simulink model "rlKinovaBallBalance"  (R2024a)
settings: Solver=ode15s  StartTime=0.0  StopTime=200  RelTol=1e-3  AbsTol=1e-3
values from neighbouring files (symbols this model uses):
  max_torque = 0.75    [kinova_params.m]
  R1_q0 = 0    [kinova_params.m]
  R4_q0 = deg2rad(135)    [kinova_params.m]
  R5_q0 = 0    [kinova_params.m]
  rover_path = rover_path1    [mars_rover_params_all.m]
  U0 = [shoulder_torque_0 elbow_torque_0 wrist_torque_0 hand_torque_0]    [kinova_params.m]
undefined symbols (not defined in the file or in its folder): ball, Control, L1, L2, L3, LS1, LS3, plate, R1, R2, R3, Rover, RS1, RS3, X, Y, Z
libraries: sm_lib x256, nesl_utility x104, fl_lib x85, nesl_utility_internal x21, sdl_lib x20, ee_lib x10, mars_rover_lib x6, simulink x3, slpidlib x2, batteryecm_lib x2, robotalgslib x1, rllib x1
(part 6 of 11)

== system rlKinovaBallBalance/Kinova Ball Balance/Rover/Terrain/Contact ==
  Contact L1 : sm_lib/Forces and Torques/Spatial Contact Force  NormalForceType=SmoothSpringDamper  NormalStiffness=contact_k  NormalStiffnessUnits=N/m  NormalDamping=contact_d  NormalDampingUnits=N/(m/s)  NormalTransitionRegionWidth=contact_tw  NormalTransitionRegionWidthUnits=m  FrictionType=SmoothStickSlip  CoefficientOfStaticFriction=friction_mus  CoefficientOfDynamicFriction=friction_mud  FrictionalCriticalVelocity=friction_vcrit  FrictionalCriticalVelocityUnits=m/s  SenseContactSignal=off  SensePenetrationDepth=off  SenseSeparationDistance=off  SenseNormalForceMagnitude=off  SenseFrictionalForceMagnitude=off  SenseNormalVelocity=off  SenseTangentialVelocity=off  SenseContactBaseRotation=off  SenseContactBaseTranslation=off  SenseContactFollowerRotation=off  SenseContactFollowerTranslation=off  ZeroCrossDetectContactStartAndEnd=off
  Contact L2 : sm_lib/Forces and Torques/Spatial Contact Force  NormalForceType=SmoothSpringDamper  NormalStiffness=contact_k  NormalStiffnessUnits=N/m  NormalDamping=contact_d  NormalDampingUnits=N/(m/s)  NormalTransitionRegionWidth=contact_tw  NormalTransitionRegionWidthUnits=m  FrictionType=SmoothStickSlip  CoefficientOfStaticFriction=friction_mus  CoefficientOfDynamicFriction=friction_mud  FrictionalCriticalVelocity=friction_vcrit  FrictionalCriticalVelocityUnits=m/s  SenseContactSignal=off  SensePenetrationDepth=off  SenseSeparationDistance=off  SenseNormalForceMagnitude=off  SenseFrictionalForceMagnitude=off  SenseNormalVelocity=off  SenseTangentialVelocity=off  SenseContactBaseRotation=off  SenseContactBaseTranslation=off  SenseContactFollowerRotation=off  SenseContactFollowerTranslation=off  ZeroCrossDetectContactStartAndEnd=off
  Contact L3 : sm_lib/Forces and Torques/Spatial Contact Force  NormalForceType=SmoothSpringDamper  NormalStiffness=contact_k  NormalStiffnessUnits=N/m  NormalDamping=contact_d  NormalDampingUnits=N/(m/s)  NormalTransitionRegionWidth=contact_tw  NormalTransitionRegionWidthUnits=m  FrictionType=SmoothStickSlip  CoefficientOfStaticFriction=friction_mus  CoefficientOfDynamicFriction=friction_mud  FrictionalCriticalVelocity=friction_vcrit  FrictionalCriticalVelocityUnits=m/s  SenseContactSignal=off  SensePenetrationDepth=off  SenseSeparationDistance=off  SenseNormalForceMagnitude=off  SenseFrictionalForceMagnitude=off  SenseNormalVelocity=off  SenseTangentialVelocity=off  SenseContactBaseRotation=off  SenseContactBaseTranslation=off  SenseContactFollowerRotation=off  SenseContactFollowerTranslation=off  ZeroCrossDetectContactStartAndEnd=off
  Contact R1 : sm_lib/Forces and Torques/Spatial Contact Force  NormalForceType=SmoothSpringDamper  NormalStiffness=contact_k  NormalStiffnessUnits=N/m  NormalDamping=contact_d  NormalDampingUnits=N/(m/s)  NormalTransitionRegionWidth=contact_tw  NormalTransitionRegionWidthUnits=m  FrictionType=SmoothStickSlip  CoefficientOfStaticFriction=friction_mus  CoefficientOfDynamicFriction=friction_mud  FrictionalCriticalVelocity=friction_vcrit  FrictionalCriticalVelocityUnits=m/s  SenseContactSignal=off  SensePenetrationDepth=off  SenseSeparationDistance=off  SenseNormalForceMagnitude=off  SenseFrictionalForceMagnitude=off  SenseNormalVelocity=off  SenseTangentialVelocity=off  SenseContactBaseRotation=off  SenseContactBaseTranslation=off  SenseContactFollowerRotation=off  SenseContactFollowerTranslation=off  ZeroCrossDetectContactStartAndEnd=off
  Contact R2 : sm_lib/Forces and Torques/Spatial Contact Force  NormalForceType=SmoothSpringDamper  NormalStiffness=contact_k  NormalStiffnessUnits=N/m  NormalDamping=contact_d  NormalDampingUnits=N/(m/s)  NormalTransitionRegionWidth=contact_tw  NormalTransitionRegionWidthUnits=m  FrictionType=SmoothStickSlip  CoefficientOfStaticFriction=friction_mus  CoefficientOfDynamicFriction=friction_mud  FrictionalCriticalVelocity=friction_vcrit  FrictionalCriticalVelocityUnits=m/s  SenseContactSignal=off  SensePenetrationDepth=off  SenseSeparationDistance=off  SenseNormalForceMagnitude=off  SenseFrictionalForceMagnitude=off  SenseNormalVelocity=off  SenseTangentialVelocity=off  SenseContactBaseRotation=off  SenseContactBaseTranslation=off  SenseContactFollowerRotation=off  SenseContactFollowerTranslation=off  ZeroCrossDetectContactStartAndEnd=off
  Contact R3 : sm_lib/Forces and Torques/Spatial Contact Force  NormalForceType=SmoothSpringDamper  NormalStiffness=contact_k  NormalStiffnessUnits=N/m  NormalDamping=contact_d  NormalDampingUnits=N/(m/s)  NormalTransitionRegionWidth=contact_tw  NormalTransitionRegionWidthUnits=m  FrictionType=SmoothStickSlip  CoefficientOfStaticFriction=friction_mus  CoefficientOfDynamicFriction=friction_mud  FrictionalCriticalVelocity=friction_vcrit  FrictionalCriticalVelocityUnits=m/s  SenseContactSignal=off  SensePenetrationDepth=off  SenseSeparationDistance=off  SenseNormalForceMagnitude=off  SenseFrictionalForceMagnitude=off  SenseNormalVelocity=off  SenseTangentialVelocity=off  SenseContactBaseRotation=off  SenseContactBaseTranslation=off  SenseContactFollowerRotation=off  SenseContactFollowerTranslation=off  ZeroCrossDetectContactStartAndEnd=off
  Simscape Bus : SimscapeBus  HierarchyStrings=L1;L2;L3;R1;R2;R3
  Wheels : PMIOPort  Side=Right
  Surface : PMIOPort  Port=2  Side=Right
  connections:
  Contact R2/RConn1 -- Simscape Bus/LConn5
  Contact L2/RConn1 -- Simscape Bus/LConn2
  Contact L1/LConn1 -- Contact L2/LConn1 -- Contact L3/LConn1 -- Surface/RConn1 -- Contact R1/LConn1 -- Contact R3/LConn1 -- Contact R2/LConn1
  Contact L1/RConn1 -- Simscape Bus/LConn1
  Contact R3/RConn1 -- Simscape Bus/LConn6
  Simscape Bus/RConn1 -- Wheels/RConn1
  Contact R1/RConn1 -- Simscape Bus/LConn4
  Contact L3/RConn1 -- Simscape Bus/LConn3

== system rlKinovaBallBalance/Kinova Ball Balance/7 DOF Manipulator/Bracelet_Link/Bracelet Link/FileSolid ==
  Bracelet Link : sm_lib/Body Elements/File Solid  ExtGeomFileName=bracelet_with_vision_link.STL  UnitType=Custom  ExtGeomFileUnits=m  StepReaderType=HEX  ExportConvexHullGeometry=off  InertiaType=Custom  BasedOnType=DensityFromFile  Density=1000  DensityUnits=kg/m^3  Mass=0.0639903  MassUnits=kg  CenterOfMass=[-0.000374733, 0.0200972, 0.0397002]  CenterOfMassUnits=m  MomentsOfInertia=[8.77763e-05, 5.386e-05, 0.000111032]  MomentsOfInertiaUnits=kg*m^2  ProductsOfInertia=[-7.81917e-06, 1.77829e-07, -4.01652e-07]  ProductsOfInertiaUnits=kg*m^2  GraphicType=FromGeometry  MarkerShape=Sphere  MarkerSize=10  GraphicVisPropType=SimpleVisualProperties  GraphicDiffuseColor=[0.6666667 0.77254903 0.92941177]  GraphicOpacity=1  GraphicSpecularColor=[0.5 0.5 0.5 1.0]  GraphicAmbientColor=[0.15 0.15 0.15 1.0]  GraphicEmissiveColor=[0.0 0.0 0.0 1.0]  GraphicShininess=75  DoExposeReferenceFrame=on  SerializedFrames=<Frames/>
  R : PMIOPort  Side=Right
  connections:
  Bracelet Link/RConn1 -- R/RConn1

== system rlKinovaBallBalance/Kinova Ball Balance/7 DOF Manipulator/Bracelet_Link/Bracelet Link/Inertia ==
  Inertia1 : sm_lib/Body Elements/Inertia  InertiaType=Custom  Mass=0.0639903  MassUnits=kg  CenterOfMass=[-0.000374733, 0.0200972, 0.0397002]  CenterOfMassUnits=m  MomentsOfInertia=[8.77763e-05, 5.386e-05, 0.000111032]  MomentsOfInertiaUnits=kg*m^2  ProductsOfInertia=[-7.81917e-06, 1.77829e-07, -4.01652e-07]  ProductsOfInertiaUnits=kg*m^2  GraphicType=Marker  MarkerShape=Inertia  MarkerSize=20  GraphicVisPropType=SimpleVisualProperties  GraphicDiffuseColor=[0.5 0.5 0.5]  GraphicOpacity=1.0  GraphicSpecularColor=[0.5 0.5 0.5 1.0]  GraphicAmbientColor=[0.15 0.15 0.15 1.0]  GraphicEmissiveColor=[0.0 0.0 0.0 1.0]  GraphicShininess=75
  R : PMIOPort  Side=Right
  connections:
  Inertia1/RConn1 -- R/RConn1

== system rlKinovaBallBalance/Kinova Ball Balance/7 DOF Manipulator/ForeArm_Link/ForeArm Link/FileSolid ==
  Forearm Link : sm_lib/Body Elements/File Solid  ExtGeomFileName=forearm_link.STL  UnitType=Custom  ExtGeomFileUnits=m  StepReaderType=HEX  ExportConvexHullGeometry=off  InertiaType=Custom  BasedOnType=DensityFromFile  Density=1000  DensityUnits=kg/m^3  Mass=0.108759  MassUnits=kg  CenterOfMass=[0.0794976, 0.0148416, -8.39544e-07]  CenterOfMassUnits=m  MomentsOfInertia=[0.000118324, 0.000832188, 0.000809477]  MomentsOfInertiaUnits=kg*m^2  ProductsOfInertia=[3.60538e-09, -2.24072e-09, 7.50733e-05]  ProductsOfInertiaUnits=kg*m^2  GraphicType=FromGeometry  MarkerShape=Sphere  MarkerSize=10  GraphicVisPropType=SimpleVisualProperties  GraphicDiffuseColor=[0.54509807 0.654902 0.77254903]  GraphicOpacity=1  GraphicSpecularColor=[0.5 0.5 0.5 1.0]  GraphicAmbientColor=[0.15 0.15 0.15 1.0]  GraphicEmissiveColor=[0.0 0.0 0.0 1.0]  GraphicShininess=75  DoExposeReferenceFrame=on  SerializedFrames=<Frames/>
  R : PMIOPort  Side=Right
  connections:
  Forearm Link/RConn1 -- R/RConn1

== system rlKinovaBallBalance/Kinova Ball Balance/7 DOF Manipulator/ForeArm_Link/ForeArm Link/Inertia ==
  Inertia1 : sm_lib/Body Elements/Inertia  InertiaType=Custom  Mass=0.108759  MassUnits=kg  CenterOfMass=[0.0794976, 0.0148416, -8.39544e-07]  CenterOfMassUnits=m  MomentsOfInertia=[0.000118324, 0.000832188, 0.000809477]  MomentsOfInertiaUnits=kg*m^2  ProductsOfInertia=[3.60538e-09, -2.24072e-09, 7.50733e-05]  ProductsOfInertiaUnits=kg*m^2  GraphicType=Marker  MarkerShape=Inertia  MarkerSize=20  GraphicVisPropType=SimpleVisualProperties  GraphicDiffuseColor=[0.5 0.5 0.5]  GraphicOpacity=1.0  GraphicSpecularColor=[0.5 0.5 0.5 1.0]  GraphicAmbientColor=[0.15 0.15 0.15 1.0]  GraphicEmissiveColor=[0.0 0.0 0.0 1.0]  GraphicShininess=75
  R : PMIOPort  Side=Right
  connections:
  Inertia1/RConn1 -- R/RConn1

== system rlKinovaBallBalance/Kinova Ball Balance/7 DOF Manipulator/HalfArm1_Link/HalfArm1 Link/FileSolid ==
  Half Arm1 Link : sm_lib/Body Elements/File Solid  ExtGeomFileName=half_arm_1_link.STL  UnitType=Custom  ExtGeomFileUnits=m  StepReaderType=HEX  ExportConvexHullGeometry=off  InertiaType=Custom  BasedOnType=DensityFromFile  Density=1000  DensityUnits=kg/m^3  Mass=0.137977  MassUnits=kg  CenterOfMass=[0.100808, 0.0121234, 4.10274e-06]  CenterOfMassUnits=m  MomentsOfInertia=[0.000202425, 0.00113112, 0.00110619]  MomentsOfInertiaUnits=kg*m^2  ProductsOfInertia=[1.72409e-08, -8.98835e-09, 0.000105223]  ProductsOfInertiaUnits=kg*m^2  GraphicType=FromGeometry  MarkerShape=Sphere  MarkerSize=10  GraphicVisPropType=SimpleVisualProperties  GraphicDiffuseColor=[0.54509807 0.654902 0.77254903]  GraphicOpacity=1  GraphicSpecularColor=[0.5 0.5 0.5 1.0]  GraphicAmbientColor=[0.15 0.15 0.15 1.0]  GraphicEmissiveColor=[0.0 0.0 0.0 1.0]  GraphicShininess=75  DoExposeReferenceFrame=on  SerializedFrames=<Frames/>
  R : PMIOPort  Side=Right
  connections:
  Half Arm1 Link/RConn1 -- R/RConn1

== system rlKinovaBallBalance/Kinova Ball Balance/7 DOF Manipulator/HalfArm1_Link/HalfArm1 Link/Inertia ==
  Inertia1 : sm_lib/Body Elements/Inertia  InertiaType=Custom  Mass=0.137977  MassUnits=kg  CenterOfMass=[0.100808, 0.0121234, 4.10274e-06]  CenterOfMassUnits=m  MomentsOfInertia=[0.000202425, 0.00113112, 0.00110619]  MomentsOfInertiaUnits=kg*m^2  ProductsOfInertia=[1.72409e-08, -8.98835e-09, 0.000105223]  ProductsOfInertiaUnits=kg*m^2  GraphicType=Marker  MarkerShape=Inertia  MarkerSize=20  GraphicVisPropType=SimpleVisualProperties  GraphicDiffuseColor=[0.5 0.5 0.5]  GraphicOpacity=1.0  GraphicSpecularColor=[0.5 0.5 0.5 1.0]  GraphicAmbientColor=[0.15 0.15 0.15 1.0]  GraphicEmissiveColor=[0.0 0.0 0.0 1.0]  GraphicShininess=75
  R : PMIOPort  Side=Right
  connections:
  Inertia1/RConn1 -- R/RConn1

== system rlKinovaBallBalance/Kinova Ball Balance/7 DOF Manipulator/HalfArm2_Link/HalfArm2 Link/FileSolid ==
  Half Arm2 Link : sm_lib/Body Elements/File Solid  ExtGeomFileName=half_arm_2_link.STL  UnitType=Custom  ExtGeomFileUnits=m  StepReaderType=HEX  ExportConvexHullGeometry=off  InertiaType=Custom  BasedOnType=DensityFromFile  Density=1000  DensityUnits=kg/m^3  Mass=0.137978  MassUnits=kg  CenterOfMass=[0.0871838, 0.0118108, 4.16659e-06]  CenterOfMassUnits=m  MomentsOfInertia=[0.000195075, 0.0011006, 0.00106833]  MomentsOfInertiaUnits=kg*m^2  ProductsOfInertia=[1.66656e-08, -1.69023e-08, 7.86653e-05]  ProductsOfInertiaUnits=kg*m^2  GraphicType=FromGeometry  MarkerShape=Sphere  MarkerSize=10  GraphicVisPropType=SimpleVisualProperties  GraphicDiffuseColor=[0.6666667 0.77254903 0.92941177]  GraphicOpacity=1  GraphicSpecularColor=[0.5 0.5 0.5 1.0]  GraphicAmbientColor=[0.15 0.15 0.15 1.0]  GraphicEmissiveColor=[0.0 0.0 0.0 1.0]  GraphicShininess=75  DoExposeReferenceFrame=on  SerializedFrames=<Frames/>
  R : PMIOPort  Side=Right
  connections:
  Half Arm2 Link/RConn1 -- R/RConn1

== system rlKinovaBallBalance/Kinova Ball Balance/7 DOF Manipulator/HalfArm2_Link/HalfArm2 Link/Inertia ==
  Inertia1 : sm_lib/Body Elements/Inertia  InertiaType=Custom  Mass=0.137978  MassUnits=kg  CenterOfMass=[0.0871838, 0.0118108, 4.16659e-06]  CenterOfMassUnits=m  MomentsOfInertia=[0.000195075, 0.0011006, 0.00106833]  MomentsOfInertiaUnits=kg*m^2  ProductsOfInertia=[1.66656e-08, -1.69023e-08, 7.86653e-05]  ProductsOfInertiaUnits=kg*m^2  GraphicType=Marker  MarkerShape=Inertia  MarkerSize=20  GraphicVisPropType=SimpleVisualProperties  GraphicDiffuseColor=[0.5 0.5 0.5]  GraphicOpacity=1.0  GraphicSpecularColor=[0.5 0.5 0.5 1.0]  GraphicAmbientColor=[0.15 0.15 0.15 1.0]  GraphicEmissiveColor=[0.0 0.0 0.0 1.0]  GraphicShininess=75
  R : PMIOPort  Side=Right
  connections:
  Inertia1/RConn1 -- R/RConn1

== system rlKinovaBallBalance/Kinova Ball Balance/7 DOF Manipulator/Shoulder_Link/Shoulder Link/FileSolid ==
  Shoulder Link : sm_lib/Body Elements/File Solid  ExtGeomFileName=shoulder_link.STL  UnitType=Custom  ExtGeomFileUnits=m  StepReaderType=HEX  ExportConvexHullGeometry=off  InertiaType=Custom  BasedOnType=DensityFromFile  Density=1000  DensityUnits=kg/m^3  Mass=0.206679  MassUnits=kg  CenterOfMass=[0.0758362, 0.0170163, 7.48345e-07]  CenterOfMassUnits=m  MomentsOfInertia=[0.000301623, 0.000658228, 0.000584422]  MomentsOfInertiaUnits=kg*m^2  ProductsOfInertia=[6.12368e-09, 4.93274e-09, -6.36892e-05]  ProductsOfInertiaUnits=kg*m^2  GraphicType=FromGeometry  MarkerShape=Sphere  MarkerSize=10  GraphicVisPropType=SimpleVisualProperties  GraphicDiffuseColor=[0.6666667 0.77254903 0.92941177]  GraphicOpacity=1  GraphicSpecularColor=[0.5 0.5 0.5 1.0]  GraphicAmbientColor=[0.15 0.15 0.15 1.0]  GraphicEmissiveColor=[0.0 0.0 0.0 1.0]  GraphicShininess=75  DoExposeReferenceFrame=on  SerializedFrames=<Frames/>
  R : PMIOPort  Side=Right
  connections:
  R/RConn1 -- Shoulder Link/RConn1

== system rlKinovaBallBalance/Kinova Ball Balance/7 DOF Manipulator/Shoulder_Link/Shoulder Link/Inertia ==
  Inertia1 : sm_lib/Body Elements/Inertia  InertiaType=Custom  Mass=0.206679  MassUnits=kg  CenterOfMass=[0.0758362, 0.0170163, 7.48345e-07]  CenterOfMassUnits=m  MomentsOfInertia=[0.000301623, 0.000658228, 0.000584422]  MomentsOfInertiaUnits=kg*m^2  ProductsOfInertia=[6.12368e-09, 4.93274e-09, -6.36892e-05]  ProductsOfInertiaUnits=kg*m^2  GraphicType=Marker  MarkerShape=Inertia  MarkerSize=20  GraphicVisPropType=SimpleVisualProperties  GraphicDiffuseColor=[0.5 0.5 0.5]  GraphicOpacity=1.0  GraphicSpecularColor=[0.5 0.5 0.5 1.0]  GraphicAmbientColor=[0.15 0.15 0.15 1.0]  GraphicEmissiveColor=[0.0 0.0 0.0 1.0]  GraphicShininess=75
  R : PMIOPort  Side=Right
  connections:
  Inertia1/RConn1 -- R/RConn1

== system rlKinovaBallBalance/Kinova Ball Balance/7 DOF Manipulator/Wrist1_Link/Wrist1 Link/FileSolid ==
  Wrist1 Link : sm_lib/Body Elements/File Solid  ExtGeomFileName=spherical_wrist_1_link.STL  UnitType=Custom  ExtGeomFileUnits=m  StepReaderType=HEX  ExportConvexHullGeometry=off  InertiaType=Custom  BasedOnType=DensityFromFile  Density=1000  DensityUnits=kg/m^3  Mass=0.0607261  MassUnits=kg  CenterOfMass=[0.0669267, 0.0134734, -3.64177e-07]  CenterOfMassUnits=m  MomentsOfInertia=[5.88928e-05, 0.000140521, 0.000138155]  MomentsOfInertiaUnits=kg*m^2  ProductsOfInertia=[2.83121e-09, 1.56006e-09, -2.20674e-05]  ProductsOfInertiaUnits=kg*m^2  GraphicType=FromGeometry  MarkerShape=Sphere  MarkerSize=10  GraphicVisPropType=SimpleVisualProperties  GraphicDiffuseColor=[0.6666667 0.77254903 0.92941177]  GraphicOpacity=1  GraphicSpecularColor=[0.5 0.5 0.5 1.0]  GraphicAmbientColor=[0.15 0.15 0.15 1.0]  GraphicEmissiveColor=[0.0 0.0 0.0 1.0]  GraphicShininess=75  DoExposeReferenceFrame=on  SerializedFrames=<Frames/>
  R : PMIOPort  Side=Right
  connections:
  Wrist1 Link/RConn1 -- R/RConn1

== system rlKinovaBallBalance/Kinova Ball Balance/7 DOF Manipulator/Wrist1_Link/Wrist1 Link/Inertia ==
  Inertia1 : sm_lib/Body Elements/Inertia  InertiaType=Custom  Mass=0.0607261  MassUnits=kg  CenterOfMass=[0.0669267, 0.0134734, -3.64177e-07]  CenterOfMassUnits=m  MomentsOfInertia=[5.88928e-05, 0.000140521, 0.000138155]  MomentsOfInertiaUnits=kg*m^2  ProductsOfInertia=[2.83121e-09, 1.56006e-09, -2.20674e-05]  ProductsOfInertiaUnits=kg*m^2  GraphicType=Marker  MarkerShape=Inertia  MarkerSize=20  GraphicVisPropType=SimpleVisualProperties  GraphicDiffuseColor=[0.5 0.5 0.5]  GraphicOpacity=1.0  GraphicSpecularColor=[0.5 0.5 0.5 1.0]  GraphicAmbientColor=[0.15 0.15 0.15 1.0]  GraphicEmissiveColor=[0.0 0.0 0.0 1.0]  GraphicShininess=75
  R : PMIOPort  Side=Right
  connections:
  Inertia1/RConn1 -- R/RConn1

== system rlKinovaBallBalance/Kinova Ball Balance/7 DOF Manipulator/Wrist2_Link/Wrist2 Link/FileSolid ==
  Wrist2 Link : sm_lib/Body Elements/File Solid  ExtGeomFileName=spherical_wrist_2_link.STL  UnitType=Custom  ExtGeomFileUnits=m  StepReaderType=HEX  ExportConvexHullGeometry=off  InertiaType=Custom  BasedOnType=DensityFromFile  Density=1000  DensityUnits=kg/m^3  Mass=0.0607235  MassUnits=kg  CenterOfMass=[0.0566892, 0.0133552, 2.07599e-07]  CenterOfMassUnits=m  MomentsOfInertia=[6.22269e-05, 0.000150545, 0.000151516]  MomentsOfInertiaUnits=kg*m^2  ProductsOfInertia=[-8.5602e-09, -1.23542e-08, -3.01223e-05]  ProductsOfInertiaUnits=kg*m^2  GraphicType=FromGeometry  MarkerShape=Sphere  MarkerSize=10  GraphicVisPropType=SimpleVisualProperties  GraphicDiffuseColor=[0.54509807 0.654902 0.77254903]  GraphicOpacity=1  GraphicSpecularColor=[0.5 0.5 0.5 1.0]  GraphicAmbientColor=[0.15 0.15 0.15 1.0]  GraphicEmissiveColor=[0.0 0.0 0.0 1.0]  GraphicShininess=75  DoExposeReferenceFrame=on  SerializedFrames=<Frames/>
  R : PMIOPort  Side=Right
  connections:
  Wrist2 Link/RConn1 -- R/RConn1

== system rlKinovaBallBalance/Kinova Ball Balance/7 DOF Manipulator/Wrist2_Link/Wrist2 Link/Inertia ==
  Inertia1 : sm_lib/Body Elements/Inertia  InertiaType=Custom  Mass=0.0607235  MassUnits=kg  CenterOfMass=[0.0566892, 0.0133552, 2.07599e-07]  CenterOfMassUnits=m  MomentsOfInertia=[6.22269e-05, 0.000150545, 0.000151516]  MomentsOfInertiaUnits=kg*m^2  ProductsOfInertia=[-8.5602e-09, -1.23542e-08, -3.01223e-05]  ProductsOfInertiaUnits=kg*m^2  GraphicType=Marker  MarkerShape=Inertia  MarkerSize=20  GraphicVisPropType=SimpleVisualProperties  GraphicDiffuseColor=[0.5 0.5 0.5]  GraphicOpacity=1.0  GraphicSpecularColor=[0.5 0.5 0.5 1.0]  GraphicAmbientColor=[0.15 0.15 0.15 1.0]  GraphicEmissiveColor=[0.0 0.0 0.0 1.0]  GraphicShininess=75
  R : PMIOPort  Side=Right
  connections:
  Inertia1/RConn1 -- R/RConn1

== system rlKinovaBallBalance/Kinova Ball Balance/7 DOF Manipulator/base_link/Base Link/FileSolid ==
  Base Link : sm_lib/Body Elements/File Solid  ExtGeomFileName=base_link.STL  UnitType=Custom  ExtGeomFileUnits=m  StepReaderType=HEX  ExportConvexHullGeometry=off  InertiaType=Custom  BasedOnType=DensityFromFile  Density=1000  DensityUnits=kg/m^3  Mass=1.06185  MassUnits=kg  CenterOfMass=[0.000712614, 0.0763467, 0.000106583]  CenterOfMassUnits=m  MomentsOfInertia=[0.00275492, 0.0011525, 0.00277912]  MomentsOfInertiaUnits=kg*m^2  ProductsOfInertia=[-1.84082e-06, 1.0557e-07, 2.81404e-05]  ProductsOfInertiaUnits=kg*m^2  GraphicType=FromGeometry  MarkerShape=Sphere  MarkerSize=10  GraphicVisPropType=SimpleVisualProperties  GraphicDiffuseColor=[0.54509807 0.654902 0.77254903]  GraphicOpacity=1  GraphicSpecularColor=[0.5 0.5 0.5 1.0]  GraphicAmbientColor=[0.15 0.15 0.15 1.0]  GraphicEmissiveColor=[0.0 0.0 0.0 1.0]  GraphicShininess=75  DoExposeReferenceFrame=on  SerializedFrames=<Frames/>
  R : PMIOPort  Side=Right
  connections:
  Base Link/RConn1 -- R/RConn1

== system rlKinovaBallBalance/Kinova Ball Balance/7 DOF Manipulator/base_link/Base Link/Inertia ==
  Inertia : sm_lib/Body Elements/Inertia  InertiaType=Custom  Mass=1.06185  MassUnits=kg  CenterOfMass=[0.000712614, 0.0763467, 0.000106583]  CenterOfMassUnits=m  MomentsOfInertia=[0.00275492, 0.0011525, 0.00277912]  MomentsOfInertiaUnits=kg*m^2  ProductsOfInertia=[-1.84082e-06, 1.0557e-07, 2.81404e-05]  ProductsOfInertiaUnits=kg*m^2  GraphicType=Marker  MarkerShape=Inertia  MarkerSize=20  GraphicVisPropType=SimpleVisualProperties  GraphicDiffuseColor=[0.5 0.5 0.5]  GraphicOpacity=1.0  GraphicSpecularColor=[0.5 0.5 0.5 1.0]  GraphicAmbientColor=[0.15 0.15 0.15 1.0]  GraphicEmissiveColor=[0.0 0.0 0.0 1.0]  GraphicShininess=75
  R : PMIOPort  Side=Right
  connections:
  Inertia/RConn1 -- R/RConn1

== system rlKinovaBallBalance/Kinova Ball Balance/Control/Chassis Control/Ackerman Steer Angle/Hold Steer at Goal ==
  d : Inport
  Enable : EnablePort
  d_h : Outport
  wires:
  d/1 -> d_h/1

== system rlKinovaBallBalance/Kinova Ball Balance/Control/Chassis Control/Steering Controller/Bus to Vec ==
  B : Inport
  Bus Selector : BusSelector  OutputSignals=q.L3,q.L1,q.R3,q.R1
  Mux : Mux
  V : Outport
  wires:
  Bus Selector/1 -> Mux/1  "<L3>"
  Bus Selector/4 -> Mux/4  "<R1>"
  Mux/1 -> V/1
  Bus Selector/2 -> Mux/2  "<L1>"
  Bus Selector/3 -> Mux/3  "<R3>"
  B/1 -> Bus Selector/1

== system rlKinovaBallBalance/Kinova Ball Balance/Control/Chassis Control/Steering Controller/Check Difference ==
  tgt : Inport
  meas : Inport  Port=2
  Demux1 : Demux
  Demux2 : Demux
  Mux{,1..3} (4 alike) : Mux  Inputs=2
  L3 : Outport
  L1 : Outport  Port=2
  R3 : Outport  Port=3
  R1 : Outport  Port=4
  wires:
  Demux2/1 -> Mux/2
  Demux1/3 -> Mux2/1
  Demux1/2 -> Mux1/1
  Demux2/4 -> Mux3/2
  Demux2/2 -> Mux1/2
  Demux2/3 -> Mux2/2
  meas/1 -> Demux2/1
  Demux1/1 -> Mux/1
  Mux1/1 -> L1/1
  Demux1/4 -> Mux3/1
  Mux3/1 -> R1/1
  Mux2/1 -> R3/1
  Mux/1 -> L3/1
  tgt/1 -> Demux1/1

== system rlKinovaBallBalance/Kinova Ball Balance/Control/Chassis Control/Steering Controller/Filter qMeas ==
  In : Inport
  Gain : Gain  Gain=1./b
  Integrator : Integrator  InitialCondition=x_initial.*b
  Sum : Sum  Inputs=|+-  InputSameDT=on  SaturateOnIntegerOverflow=on  OutDataTypeStr=Inherit: Same as first input
  Out : Outport  VectorParamsAs1DForOutWhenUnconnected=off
  wires:
  Sum/1 -> Integrator/1
  In/1 -> Sum/1
  Integrator/1 -> Gain/1
  Gain/1 -> Sum/2, Out/1

== system rlKinovaBallBalance/Kinova Ball Balance/Control/Chassis Control/Steering Controller/Filter qTarget ==
  In : Inport
  Gain : Gain  Gain=1./b
  Integrator : Integrator  InitialCondition=x_initial.*b
  Sum : Sum  Inputs=|+-  InputSameDT=on  SaturateOnIntegerOverflow=on  OutDataTypeStr=Inherit: Same as first input
  Out : Outport  VectorParamsAs1DForOutWhenUnconnected=off
  wires:
  Gain/1 -> Out/1, Sum/2
  Integrator/1 -> Gain/1
  In/1 -> Sum/1
  Sum/1 -> Integrator/1

== system rlKinovaBallBalance/Kinova Ball Balance/Control/Chassis Control/Target Direction and Speed/Check Distance To Goal ==
  note: Distance from Goal to satisfy that the robot has reached the goal
  goal : Inport
  currentPose : Inport  Port=2
  linVel : Inport  Port=3
  Add : Sum
  Constant : Constant  Value=0.25
  Constant1 : Constant  Value=2*Control.Drive.TargetAccel
  Divide : Product  Inputs=*/
  Dot Product : DotProduct  OutDataTypeStr=Inherit: Inherit via internal rule
  Gain1 : Gain
  Less Than : RelationalOperator  Operator=>  OutDataTypeStr=boolean  RndMeth=Simplest  InputSameDT=off
  Less Than1 : RelationalOperator  Operator=>  OutDataTypeStr=boolean  RndMeth=Simplest  InputSameDT=off
  NOT : Logic  Operator=NOT  IconShape=distinctive  AllPortsSameDT=off  OutDataTypeStr=boolean
  Scope1 : Scope
  Selector : Selector  InputPortWidth=3  IndexOptions=Index vector (dialog)  Indices=[1 2]  OutputSizes=1
  Sqrt : Sqrt
  Subtract : Sum  Inputs=+-
  Unit Delay : UnitDelay  SampleTime=-1  HasFrameUpgradeWarning=on
  const : Math  Operator=square
  atGoal : Outport
  Slow : Outport  Port=2
  wires:
  goal/1 -> Subtract/2
  Dot Product/1 -> Sqrt/1
  Constant/1 -> Gain1/1, Less Than/2
  currentPose/1 -> Selector/1
  Sqrt/1 -> Scope1/1, Less Than/1, Less Than1/1
  Subtract/1 -> Dot Product/2, Dot Product/1
  Selector/1 -> Subtract/1
  linVel/1 -> const/1
  const/1 -> Divide/1
  Constant1/1 -> Divide/2
  Less Than1/1 -> Slow/1
  Add/1 -> Less Than1/2
  Divide/1 -> Add/1
  Gain1/1 -> Add/2
  Less Than/1 -> NOT/1
  NOT/1 -> Unit Delay/1
  Unit Delay/1 -> atGoal/1

== system rlKinovaBallBalance/Kinova Ball Balance/Control/Chassis Control/Target Direction and Speed/hold ==
  In1 : Inport
  Constant9 : Constant  Value=inf
  NOT1 : Logic  Operator=NOT  IconShape=distinctive  AllPortsSameDT=off  OutDataTypeStr=boolean
  RoverStopTime : Subsystem
  Switch3 : Switch  Criteria=u2 > Threshold  SaturateOnIntegerOverflow=off  InputSameDT=off
  Unit Delay1 : UnitDelay  SampleTime=-1  HasFrameUpgradeWarning=on
  Out1 : Outport
  wires:
  Unit Delay1/1 -> Switch3/2
  RoverStopTime/1(DeAccelTime) -> Switch3/1
  Switch3/1 -> Out1/1
  NOT1/1 -> RoverStopTime/1(Enable), Unit Delay1/1
  Constant9/1 -> Switch3/3
  In1/1 -> NOT1/1

== system rlKinovaBallBalance/Kinova Ball Balance/Control/Chassis Control/Wheel Speed Controller/Bus to Vec ==
  B : Inport
  Bus Selector : BusSelector  OutputSignals=w.L1,w.L2,w.L3,w.R1,w.R2,w.R3
  Mux : Mux  Inputs=6
  V : Outport
  wires:
  Bus Selector/1 -> Mux/1  "<L1>"
  Bus Selector/3 -> Mux/3  "<L3>"
  Bus Selector/4 -> Mux/4  "<R1>"
  Bus Selector/6 -> Mux/6  "<R3>"
  Bus Selector/5 -> Mux/5  "<R2>"
  Bus Selector/2 -> Mux/2  "<L2>"
  B/1 -> Bus Selector/1
  Mux/1 -> V/1

== system rlKinovaBallBalance/Kinova Ball Balance/Control/Chassis Control/Wheel Speed Controller/Filter wMeas ==
  In : Inport
  Gain : Gain  Gain=1./b
  Integrator : Integrator  InitialCondition=x_initial.*b
  Sum : Sum  Inputs=|+-  InputSameDT=on  SaturateOnIntegerOverflow=on  OutDataTypeStr=Inherit: Same as first input
  Out : Outport  VectorParamsAs1DForOutWhenUnconnected=off
  wires:
  Sum/1 -> Integrator/1
  In/1 -> Sum/1
  Integrator/1 -> Gain/1
  Gain/1 -> Sum/2, Out/1

== system rlKinovaBallBalance/Kinova Ball Balance/Control/Chassis Control/Wheel Speed Controller/Filter wTarget ==
  In : Inport
  Gain : Gain  Gain=1./b
  Integrator : Integrator  InitialCondition=x_initial.*b
  Sum : Sum  Inputs=|+-  InputSameDT=on  SaturateOnIntegerOverflow=on  OutDataTypeStr=Inherit: Same as first input
  Out : Outport  VectorParamsAs1DForOutWhenUnconnected=off
  wires:
  Gain/1 -> Out/1, Sum/2
  Integrator/1 -> Gain/1
  In/1 -> Sum/1
  Sum/1 -> Integrator/1

== system rlKinovaBallBalance/Kinova Ball Balance/Rover/Chassis/Camera/rsm_base_1_RIGID ==
  ReferenceFrame : sm_lib/Frames and Transforms/Reference Frame
  Solid : sm_lib/Body Elements/File Solid  ExtGeomFileName=rover_chassis_sensor_base.stl  UnitType=Custom  ExtGeomFileUnits=cm  StepReaderType=HEX  ExportConvexHullGeometry=off  InertiaType=CalculateFromGeometry  BasedOnType=Density  Density=2000  DensityUnits=kg/m^3  Mass=202690.508551217  MassUnits=kg  CenterOfMass=[-2.09994238818055e-07 21.8231915316941 -2.20167989735098e-07]  CenterOfMassUnits=m  MomentsOfInertia=[2411866.97125594 5940029.20050206 6701187.74240286]  MomentsOfInertiaUnits=kg*m^2  ProductsOfInertia=[0.00792234309140369 -0.0164088810985133 -0.460936358460458]  ProductsOfInertiaUnits=kg*m^2  GraphicType=FromGeometry  MarkerShape=Sphere  MarkerSize=10  GraphicVisPropType=SimpleVisualProperties  GraphicDiffuseColor=[0.2 0.2 0.2]  GraphicOpacity=1  GraphicSpecularColor=[0.5 0.5 0.5 1.0]  GraphicAmbientColor=[0.15 0.15 0.15 1.0]  GraphicEmissiveColor=[0.0 0.0 0.0 1.0]  GraphicShininess=75  DoExposeReferenceFrame=on  SerializedFrames=<Frames/>
  Transform : sm_lib/Frames and Transforms/Rigid Transform  RotationMethod=ArbitraryAxis  FollAlignAxisA=+X  BaseAlignAxisA=+Y  FollAlignAxisB=+Y  BaseAlignAxisB=+Z  RotationStandardAxis=+Z  RotationAngle=2.0943951023932  RotationAngleUnits=rad  RotationArbitraryAxis=[0.577350269189626 0.577350269189626 0.577350269189626]  RotationSequenceAxes=FollowerAxes  RotationSequence=XYX  RotationSequenceAngles=[0 0 0]  RotationSequenceAnglesUnits=deg  RotationMatrix=[1 0 0; 0 1 0; 0 0 1]  Quaternion=[1 0 0 0]  TranslationMethod=Cartesian  TranslationCartesianOffset=[-40 220.000003786473 -2.05636384635e-06]  TranslationCartesianOffsetUnits=mm  TranslationStandardAxis=+Z  TranslationStandardOffset=0  TranslationStandardOffsetUnits=mm  TranslationROffset=0  TranslationROffsetUnits=m  TranslationThetaOffset=0  TranslationThetaOffsetUnits=deg  TranslationZOffset=0  TranslationZOffsetUnits=m
  F : PMIOPort  Side=Right
  F1 : PMIOPort  Port=2  Side=Left
  connections:
  Transform/LConn1 -- F1/RConn1 -- ReferenceFrame/RConn1 -- Solid/RConn1
  Transform/RConn1 -- F/RConn1

== system rlKinovaBallBalance/Kinova Ball Balance/Rover/Chassis/Camera/rsm_head_1_RIGID ==
  Reference Camera : sm_lib/Frames and Transforms/Reference Frame
  ReferenceFrame : sm_lib/Frames and Transforms/Reference Frame
  Rigid Transform : sm_lib/Frames and Transforms/Rigid Transform  RotationMethod=StandardAxis  FollAlignAxisA=+X  BaseAlignAxisA=+Y  FollAlignAxisB=+Y  BaseAlignAxisB=+Z  RotationStandardAxis=+X  RotationAngle=-90  RotationAngleUnits=deg  RotationArbitraryAxis=[0 0 1]  RotationSequenceAxes=FollowerAxes  RotationSequence=XYX  RotationSequenceAngles=[0 0 0]  RotationSequenceAnglesUnits=deg  RotationMatrix=[1 0 0; 0 1 0; 0 0 1]  Quaternion=[1 0 0 0]  TranslationMethod=Cartesian  TranslationCartesianOffset=[12 11 13]  TranslationCartesianOffsetUnits=cm  TranslationStandardAxis=+Z  TranslationStandardOffset=0  TranslationStandardOffsetUnits=cm  TranslationROffset=0  TranslationROffsetUnits=m  TranslationThetaOffset=0  TranslationThetaOffsetUnits=deg  TranslationZOffset=0  TranslationZOffsetUnits=m
  Solid : sm_lib/Body Elements/File Solid  ExtGeomFileName=rover_chassis_sensor_head.stl  UnitType=Custom  ExtGeomFileUnits=cm  StepReaderType=HEX  ExportConvexHullGeometry=off  InertiaType=CalculateFromGeometry  BasedOnType=Density  Density=2000  DensityUnits=kg/m^3  Mass=1  MassUnits=kg  CenterOfMass=[-0.00288550161429388 71.0000014663329 -4.54954138701768e-07]  CenterOfMassUnits=m  MomentsOfInertia=[1608495.92335293 6519098.97331966 6519098.97331985]  MomentsOfInertiaUnits=kg*m^2  ProductsOfInertia=[-6.49609544482223e-08 0.336731288221059 1.08955853960892]  ProductsOfInertiaUnits=kg*m^2  GraphicType=FromGeometry  MarkerShape=Sphere  MarkerSize=10  GraphicVisPropType=SimpleVisualProperties  GraphicDiffuseColor=[0.80784315 0.80784315 0.6431373]  GraphicOpacity=1  GraphicSpecularColor=[1 1 1 1.0]  GraphicAmbientColor=[0.15 0.15 0.15 0.8]  GraphicEmissiveColor=[0 0 0 1]  GraphicShininess=90  DoExposeReferenceFrame=on  SerializedFrames=<Frames/>
  Transform : sm_lib/Frames and Transforms/Rigid Transform  RotationMethod=ArbitraryAxis  FollAlignAxisA=+X  BaseAlignAxisA=+Y  FollAlignAxisB=+Y  BaseAlignAxisB=+Z  RotationStandardAxis=+Z  RotationAngle=2.0943951023932  RotationAngleUnits=rad  RotationArbitraryAxis=[0.577350269189626 0.577350269189626 0.577350269189626]  RotationSequenceAxes=FollowerAxes  RotationSequence=XYX  RotationSequenceAngles=[0 0 0]  RotationSequenceAnglesUnits=deg  RotationMatrix=[1 0 0; 0 1 0; 0 0 1]  Quaternion=[1 0 0 0]  TranslationMethod=Cartesian  TranslationCartesianOffset=[-40.5288600921631 710.000004438766 -7.70947271803379e-06]  TranslationCartesianOffsetUnits=mm  TranslationStandardAxis=+Z  TranslationStandardOffset=0  TranslationStandardOffsetUnits=mm  TranslationROffset=0  TranslationROffsetUnits=m  TranslationThetaOffset=0  TranslationThetaOffsetUnits=deg  TranslationZOffset=0  TranslationZOffsetUnits=m
  F : PMIOPort  Side=Left
  connections:
  ReferenceFrame/RConn1 -- Solid/RConn1 -- Transform/LConn1
  Transform/RConn1 -- F/RConn1 -- Rigid Transform/LConn1
  Rigid Transform/RConn1 -- Reference Camera/RConn1

== system rlKinovaBallBalance/Kinova Ball Balance/Rover/Chassis/Camera/rsm_lower_mast_2_RIGID ==
  ReferenceFrame : sm_lib/Frames and Transforms/Reference Frame
  Solid : sm_lib/Body Elements/File Solid  ExtGeomFileName=rover_chassis_sensor_mast_lower.stl  UnitType=Custom  ExtGeomFileUnits=cm  StepReaderType=HEX  ExportConvexHullGeometry=off  InertiaType=CalculateFromGeometry  BasedOnType=Density  Density=2000  DensityUnits=kg/m^3  Mass=403410.668072862  MassUnits=kg  CenterOfMass=[4.00000000041938 10.1119460218271 35.0000011171366]  CenterOfMassUnits=m  MomentsOfInertia=[4810006.95412572 3779509.77447628 5346172.06825756]  MomentsOfInertiaUnits=kg*m^2  ProductsOfInertia=[0.0256104910578052 9.59441184474277e-11 -0.00591852250388119]  ProductsOfInertiaUnits=kg*m^2  GraphicType=FromGeometry  MarkerShape=Sphere  MarkerSize=10  GraphicVisPropType=SimpleVisualProperties  GraphicDiffuseColor=[1 1 0.8]  GraphicOpacity=1  GraphicSpecularColor=[0.5 0.5 0.5 1.0]  GraphicAmbientColor=[0.15 0.15 0.15 1.0]  GraphicEmissiveColor=[0.0 0.0 0.0 1.0]  GraphicShininess=75  DoExposeReferenceFrame=on  SerializedFrames=<Frames/>
  Transform : sm_lib/Frames and Transforms/Rigid Transform  RotationMethod=ArbitraryAxis  FollAlignAxisA=+X  BaseAlignAxisA=+Y  FollAlignAxisB=+Y  BaseAlignAxisB=+Z  RotationStandardAxis=+Z  RotationAngle=2.0943951023932  RotationAngleUnits=rad  RotationArbitraryAxis=[-0.577350269189626 -0.577350269189626 -0.577350269189626]  RotationSequenceAxes=FollowerAxes  RotationSequence=XYX  RotationSequenceAngles=[0 0 0]  RotationSequenceAnglesUnits=deg  RotationMatrix=[1 0 0; 0 1 0; 0 0 1]  Quaternion=[1 0 0 0]  TranslationMethod=Cartesian  TranslationCartesianOffset=[40.0000013147577 450.900022888183 350.000005500325]  TranslationCartesianOffsetUnits=mm  TranslationStandardAxis=+Z  TranslationStandardOffset=0  TranslationStandardOffsetUnits=mm  TranslationROffset=0  TranslationROffsetUnits=m  TranslationThetaOffset=0  TranslationThetaOffsetUnits=deg  TranslationZOffset=0  TranslationZOffsetUnits=m
  Transform1 : sm_lib/Frames and Transforms/Rigid Transform  RotationMethod=ArbitraryAxis  FollAlignAxisA=+X  BaseAlignAxisA=+Y  FollAlignAxisB=+Y  BaseAlignAxisB=+Z  RotationStandardAxis=+Z  RotationAngle=2.0943951023932  RotationAngleUnits=rad  RotationArbitraryAxis=[0.577350269189626 0.577350269189626 0.577350269189626]  RotationSequenceAxes=FollowerAxes  RotationSequence=XYX  RotationSequenceAngles=[0 0 0]  RotationSequenceAnglesUnits=deg  RotationMatrix=[1 0 0; 0 1 0; 0 0 1]  Quaternion=[1 0 0 0]  TranslationMethod=Cartesian  TranslationCartesianOffset=[0 100.000002423247 350.000011189513]  TranslationCartesianOffsetUnits=mm  TranslationStandardAxis=+Z  TranslationStandardOffset=0  TranslationStandardOffsetUnits=mm  TranslationROffset=0  TranslationROffsetUnits=m  TranslationThetaOffset=0  TranslationThetaOffsetUnits=deg  TranslationZOffset=0  TranslationZOffsetUnits=m
  F1 : PMIOPort  Side=Left
  F : PMIOPort  Port=2  Side=Right
  connections:
  Transform/LConn1 -- Transform1/LConn1 -- ReferenceFrame/RConn1 -- Solid/RConn1
  Transform/RConn1 -- F/RConn1
  Transform1/RConn1 -- F1/RConn1

== system rlKinovaBallBalance/Kinova Ball Balance/Rover/Chassis/Camera/rsm_outer_ring_1_RIGID ==
  ReferenceFrame : sm_lib/Frames and Transforms/Reference Frame
  Rigid Transform : sm_lib/Frames and Transforms/Rigid Transform  RotationMethod=StandardAxis  FollAlignAxisA=+X  BaseAlignAxisA=+Y  FollAlignAxisB=+Y  BaseAlignAxisB=+Z  RotationStandardAxis=+Z  RotationAngle=20.0  RotationAngleUnits=deg  RotationArbitraryAxis=[0 0 1]  RotationSequenceAxes=FollowerAxes  RotationSequence=XYX  RotationSequenceAngles=[0 0 0]  RotationSequenceAnglesUnits=deg  RotationMatrix=[1 0 0; 0 1 0; 0 0 1]  Quaternion=[1 0 0 0]  TranslationMethod=None  TranslationCartesianOffset=[0 0 0]  TranslationCartesianOffsetUnits=m  TranslationStandardAxis=+Z  TranslationStandardOffset=0  TranslationStandardOffsetUnits=m  TranslationROffset=0  TranslationROffsetUnits=m  TranslationThetaOffset=0  TranslationThetaOffsetUnits=deg  TranslationZOffset=0  TranslationZOffsetUnits=m
  Solid : sm_lib/Body Elements/File Solid  ExtGeomFileName=rover_chassis_sensor_ring_outer.stl  UnitType=Custom  ExtGeomFileUnits=cm  StepReaderType=HEX  ExportConvexHullGeometry=off  InertiaType=CalculateFromGeometry  BasedOnType=Density  Density=2000  DensityUnits=kg/m^3  Mass=2000  MassUnits=kg  CenterOfMass=[3.99999986837507 43.0793255522792 35.0000003648552]  CenterOfMassUnits=m  MomentsOfInertia=[35996.0863503472 57529.9697773705 35996.0863503472]  MomentsOfInertiaUnits=kg*m^2  ProductsOfInertia=[0.000493832044278217 -4.64395705120422e-11 0.00068000513182705]  ProductsOfInertiaUnits=kg*m^2  GraphicType=FromGeometry  MarkerShape=Sphere  MarkerSize=10  GraphicVisPropType=SimpleVisualProperties  GraphicDiffuseColor=[0.2 0.2 0.2]  GraphicOpacity=1  GraphicSpecularColor=[0.5 0.5 0.5 1.0]  GraphicAmbientColor=[0.15 0.15 0.15 1.0]  GraphicEmissiveColor=[0.0 0.0 0.0 1.0]  GraphicShininess=75  DoExposeReferenceFrame=on  SerializedFrames=<Frames/>
  Transform : sm_lib/Frames and Transforms/Rigid Transform  RotationMethod=ArbitraryAxis  FollAlignAxisA=+X  BaseAlignAxisA=+Y  FollAlignAxisB=+Y  BaseAlignAxisB=+Z  RotationStandardAxis=+Z  RotationAngle=2.09439510239319  RotationAngleUnits=rad  RotationArbitraryAxis=[-0.577350269189626 -0.577350269189627 -0.577350269189625]  RotationSequenceAxes=FollowerAxes  RotationSequence=XYX  RotationSequenceAngles=[0 0 0]  RotationSequenceAnglesUnits=deg  RotationMatrix=[1 0 0; 0 1 0; 0 0 1]  Quaternion=[1 0 0 0]  TranslationMethod=Cartesian  TranslationCartesianOffset=[39.9999957537947 420.900022888184 350.000001520764]  TranslationCartesianOffsetUnits=mm  TranslationStandardAxis=+Z  TranslationStandardOffset=0  TranslationStandardOffsetUnits=mm  TranslationROffset=0  TranslationROffsetUnits=m  TranslationThetaOffset=0  TranslationThetaOffsetUnits=deg  TranslationZOffset=0  TranslationZOffsetUnits=m
  Transform1 : sm_lib/Frames and Transforms/Rigid Transform  RotationMethod=ArbitraryAxis  FollAlignAxisA=+X  BaseAlignAxisA=+Y  FollAlignAxisB=+Y  BaseAlignAxisB=+Z  RotationStandardAxis=+Z  RotationAngle=2.29441736937637  RotationAngleUnits=rad  RotationArbitraryAxis=[-0.450882585021863 -0.631151683244211 -0.631151683244211]  RotationSequenceAxes=FollowerAxes  RotationSequence=XYX  RotationSequenceAngles=[0 0 0]  RotationSequenceAnglesUnits=deg  RotationMatrix=[1 0 0; 0 1 0; 0 0 1]  Quaternion=[1 0 0 0]  TranslationMethod=Cartesian  TranslationCartesianOffset=[39.9999957537972 461.900007629394 350.000001520762]  TranslationCartesianOffsetUnits=mm  TranslationStandardAxis=+Z  TranslationStandardOffset=0  TranslationStandardOffsetUnits=mm  TranslationROffset=0  TranslationROffsetUnits=m  TranslationThetaOffset=0  TranslationThetaOffsetUnits=deg  TranslationZOffset=0  TranslationZOffsetUnits=m
  F1 : PMIOPort  Side=Left
  F : PMIOPort  Port=2  Side=Left
  connections:
  Transform/LConn1 -- Transform1/LConn1 -- ReferenceFrame/RConn1 -- Solid/RConn1
  Transform/RConn1 -- F/RConn1
  Rigid Transform/RConn1 -- F1/RConn1
  Rigid Transform/LConn1 -- Transform1/RConn1

== system rlKinovaBallBalance/Kinova Ball Balance/Rover/Chassis/Camera/rsm_upper_mast_1_RIGID ==
  ReferenceFrame : sm_lib/Frames and Transforms/Reference Frame
  Solid : sm_lib/Body Elements/File Solid  ExtGeomFileName=rover_chassis_sensor_mast_upper.stl  UnitType=Custom  ExtGeomFileUnits=cm  StepReaderType=HEX  ExportConvexHullGeometry=off  InertiaType=CalculateFromGeometry  BasedOnType=Density  Density=2000  DensityUnits=kg/m^3  Mass=382776.497765057  MassUnits=kg  CenterOfMass=[3.99998590581562 58.9787952931336 34.9999786232352]  CenterOfMassUnits=m  MomentsOfInertia=[3038949.11550358 3496444.12832479 3624138.33109519]  MomentsOfInertiaUnits=kg*m^2  ProductsOfInertia=[-149.383305940768 -0.0992863146641867 -86.2313374210248]  ProductsOfInertiaUnits=kg*m^2  GraphicType=FromGeometry  MarkerShape=Sphere  MarkerSize=10  GraphicVisPropType=SimpleVisualProperties  GraphicDiffuseColor=[1 1 0.8]  GraphicOpacity=1  GraphicSpecularColor=[0.5 0.5 0.5 1.0]  GraphicAmbientColor=[0.15 0.15 0.15 1.0]  GraphicEmissiveColor=[0.0 0.0 0.0 1.0]  GraphicShininess=75  DoExposeReferenceFrame=on  SerializedFrames=<Frames/>
  Transform : sm_lib/Frames and Transforms/Rigid Transform  RotationMethod=ArbitraryAxis  FollAlignAxisA=+X  BaseAlignAxisA=+Y  FollAlignAxisB=+Y  BaseAlignAxisB=+Z  RotationStandardAxis=+Z  RotationAngle=2.0943951023932  RotationAngleUnits=rad  RotationArbitraryAxis=[-0.577350269189626 -0.577350269189626 -0.577350269189626]  RotationSequenceAxes=FollowerAxes  RotationSequence=XYX  RotationSequenceAngles=[0 0 0]  RotationSequenceAnglesUnits=deg  RotationMatrix=[1 0 0; 0 1 0; 0 0 1]  Quaternion=[1 0 0 0]  TranslationMethod=Cartesian  TranslationCartesianOffset=[39.8936241533249 429.9 349.815749642353]  TranslationCartesianOffsetUnits=mm  TranslationStandardAxis=+Z  TranslationStandardOffset=0  TranslationStandardOffsetUnits=mm  TranslationROffset=0  TranslationROffsetUnits=m  TranslationThetaOffset=0  TranslationThetaOffsetUnits=deg  TranslationZOffset=0  TranslationZOffsetUnits=m
  Transform1 : sm_lib/Frames and Transforms/Rigid Transform  RotationMethod=ArbitraryAxis  FollAlignAxisA=+X  BaseAlignAxisA=+Y  FollAlignAxisB=+Y  BaseAlignAxisB=+Z  RotationStandardAxis=+Z  RotationAngle=2.0943951023932  RotationAngleUnits=rad  RotationArbitraryAxis=[0.577350269189626 0.577350269189626 0.577350269189626]  RotationSequenceAxes=FollowerAxes  RotationSequence=XYX  RotationSequenceAngles=[0 0 0]  RotationSequenceAnglesUnits=deg  RotationMatrix=[1 0 0; 0 1 0; 0 0 1]  Quaternion=[1 0 0 0]  TranslationMethod=Cartesian  TranslationCartesianOffset=[7.105427357601e-14 590.000009936775 350.000030393688]  TranslationCartesianOffsetUnits=mm  TranslationStandardAxis=+Z  TranslationStandardOffset=0  TranslationStandardOffsetUnits=mm  TranslationROffset=0  TranslationROffsetUnits=m  TranslationThetaOffset=0  TranslationThetaOffsetUnits=deg  TranslationZOffset=0  TranslationZOffsetUnits=m
  F : PMIOPort  Side=Left
  F1 : PMIOPort  Port=2  Side=Right
  connections:
  Transform/LConn1 -- Transform1/LConn1 -- ReferenceFrame/RConn1 -- Solid/RConn1
  Transform/RConn1 -- F/RConn1
  Transform1/RConn1 -- F1/RConn1
